simulink model "prac3simu"  (R2022b)
settings: Solver=VariableStepAuto  StartTime=0.0  StopTime=10.0  RelTol=1e-3
values from neighbouring files (symbols this model uses):
  b1 = 1000    [Practica3.m]    (also in parametrosprac3.m)
  f = 0    [Practica3.m]    (also in parametrosprac3.m)
  k1 = 16182    [Practica3.m]    (also in parametrosprac3.m)
  k2 = 19000    [Practica3.m]    (also in parametrosprac3.m)
  m1 = 290    [Practica3.m]    (also in parametrosprac3.m)
  m2 = 59    [Practica3.m]    (also in parametrosprac3.m)
settings Model: Creator=52466  LastModifiedBy=52466

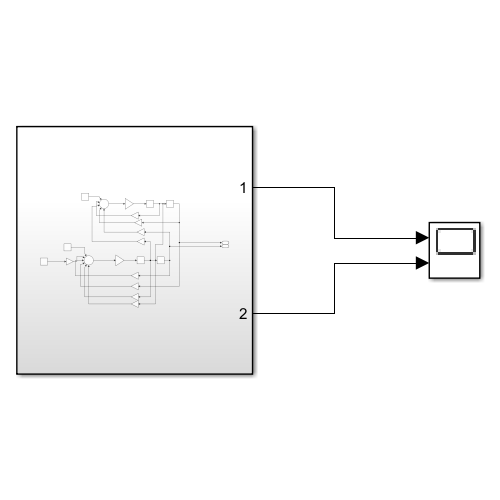
[thumbnail: Simulink's stored preview of the top-level diagram]
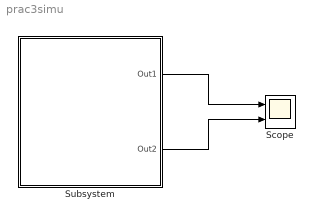
== system prac3simu ==
  Scope : Scope  NumInputPorts=2
  Subsystem : Subsystem
  wires:
  Subsystem/1(Out1) -> Scope/1
  Subsystem/2(Out2) -> Scope/2

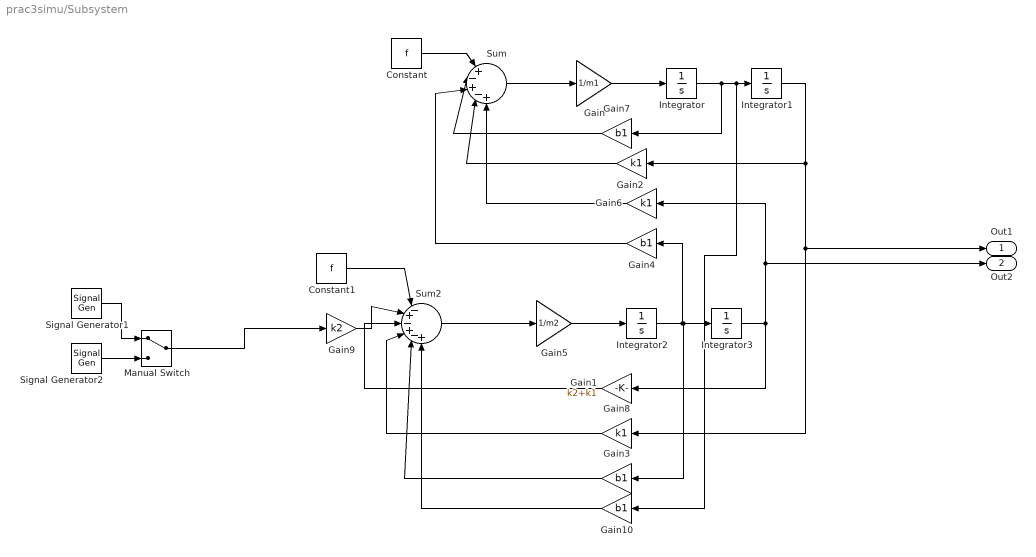
== system prac3simu/Subsystem ==
  Constant : Constant  Value=f
  Constant1 : Constant  Value=f
  Gain : Gain  Gain=1/m1
  Gain1 : Gain  Gain=k2+k1
  Gain{3..4,7,10} (4 alike) : Gain  Gain=b1
  Gain2 : Gain  Gain=k1
  Gain5 : Gain  Gain=1/m2
  Gain6 : Gain  Gain=k1
  Gain8 : Gain  Gain=k1
  Gain9 : Gain  Gain=k2
  Integrator{,1..3} (4 alike) : Integrator
  Manual Switch : ManualSwitch
  Signal Generator1 : SignalGenerator  Amplitude=0.05  Frequency=0.5*pi  Units=rad/sec
  Signal Generator2 : SignalGenerator  Amplitude=0.05  Frequency=20*pi  Units=rad/sec
  Sum : Sum  Inputs=|+-+-+
  Sum2 : Sum  Inputs=|-+-+-+
  Out1 : Outport
  Out2 : Outport  Port=2
  wires:
  Gain5/1 -> Integrator2/1
  Integrator2/1 -> Gain4/1, Gain3/1, Integrator3/1
  Gain1/1 -> Sum2/3
  Manual Switch/1 -> Gain9/1
  Gain9/1 -> Sum2/2
  Gain10/1 -> Sum2/6
  Gain4/1 -> Sum/3
  Integrator/1 -> Gain7/1, Gain10/1, Integrator1/1
  Sum2/1 -> Gain5/1
  Gain3/1 -> Sum2/5
  Gain7/1 -> Sum/2
  Integrator1/1 -> Out1/1, Gain8/1, Gain2/1
  Constant1/1 -> Sum2/1
  Sum/1 -> Gain/1
  Gain2/1 -> Sum/4
  Gain/1 -> Integrator/1
  Gain6/1 -> Sum/5
  Integrator3/1 -> Out2/1, Gain6/1, Gain1/1
  Gain8/1 -> Sum2/4
  Constant/1 -> Sum/1
  Signal Generator2/1 -> Manual Switch/2
  Signal Generator1/1 -> Manual Switch/1
